simulink library "HANcoder_STM32_Target"  (R2018a)
settings: Solver=ode45  StartTime=0.0  StopTime=10.0  RelTol=1e-3  EnableMultiTasking=on
libraries: simulink x3
(part 3 of 7)

== system HANcoder_STM32_Target/STM32-E407/SPI ==
  SPI master init : Subsystem  Tag=HANcoder_TARGET_STM32_E407  mask(SPI master init){channel=SPI1: D13 & D12 & D11, speed=5250 kHz, polarity=Idle low, phase=Sample bit on 1st clock edge}
      mask prompts: speed "Communication speed"
      mask help:
      | Function
      | ==========
      | Initialized a SPI master channel.
      |
      | Parameters per channel
      | ======================
      | - Select channel
      | - Select communication speed
      | - Select clock signal polarity
      | - Select clock phase to sample a bit
      mask init:
      | spiChannelInfoStr = sfcn_spi_master_init_mcb(2, channel, speed, polarity, phase);
      settings: CopyFcn=sfcn_spi_master_init_chk();  MoveFcn=drawLogos
      mask Help: web('sfcn_spi_master_init.html')
      mask TypeOptions channel: SPI1: D13 & D12 & D11 | SPI2: UEXT 9 & 7 & 8
      mask Callback channel: sfcn_spi_master_init_chk();
      mask TypeOptions speed: 21000 kHz | 10500 kHz | 5250 kHz | 2625 kHz | 1312.5 kHz | 656.25 kHz | 328.125 kHz | 164.0625 kHz
      mask TypeOptions polarity: Idle low | Idle high
      mask TypeOptions phase: Sample bit on 1st clock edge | Sample bit on 2nd clock edge
      mask Display: fprintf('SPI master init\n%s', spiChannelInfoStr);patch([211 217 217],[8 14 2],[1 0 0]);patch([219 219 225],[14 2 8],[0 0 0.35]);
  SPI master transfer : Subsystem  Tag=HANcoder_TARGET_STM32_E407  mask(SPI master transfer){channel=SPI1: D13 & D12 & D11, useSS=off, SSpin=CON2 - A0, SSenable=on, SSdisable=on, delayCycles=0, tsamp=-1}
      mask prompts: useSS "Use slave select output"; SSpin "Slave select output pin"; SSenable "Enable slave select before transfer"; SSdisable "Disable slave select after transfer"; delayCycles "Delay cycles between slave select enable and transfer"; tsamp "Sample time"
      mask help:
      | Function
      | ==========
      | Performs a byte transfer via SPI.
      |
      | Parameters per channel
      | ======================
      | - Select channel
      | - Select if a Slave Select output should be controlled
      |   * Select the Slave Select digital output pin
      |   * Select if the Slave Select should be made logic low before the transfer
      |   * Select if the Slave Select should be made logic high after the transfer
      |   * Enter the number of CPU cycles to delay between Slave Select enable and the transfer
      |
      | Inputs
      | ======
      | The byte value to send to the slave.
      |
      | Outputs
      | =======
      | The byte value received from the slave.
      mask init:
      | spiChannelInfoStr = sfcn_spi_master_transfer_mcb(2, channel, useSS, SSpin, SSenable, SSdisable, delayCycles);
      settings: MoveFcn=drawLogos
      mask Help: web('sfcn_spi_master_transfer.html')
      mask TypeOptions channel: SPI1: D13 & D12 & D11 | SPI2: UEXT 9 & 7 & 8
      mask TypeOptions SSpin: CON2 - A0 | CON2 - A1 | CON2 - A2 | CON2 - A3 | CON2 - A4 | CON2 - A5 | CON3 - D0 | CON3 - D1 | CON3 - D2 | CON3 - D3 | CON3 - D4 | CON3 - D5 | CON3 - D6 | CON3 - D7 | CON4 - D8 | CON4 - D9 | CON4 - D10 | CON4 - D11 | CON4 - D12 | CON4 - D13 | CON PD - 3 | CON PD - 4 | CON PD - 5 | CON PD - 6 | CON PD - 7 | CON PD - 8 | CON PD - 9 | CON PD - 10 | CON PD - 11 | CON PD - 12 | CON PD - 13 | CON PD - 14 | CON PD - 15 | CON PD - 16 | CON PD - 17 | CON PD - 18 | CON PE - 3 | CON PE - 4 | CON PE - 6 | CON PE - 10 | CON PE - 11 | CON PE - 12 | CON PE - 13 | CON PE - 14 | CON PE - 15 | CON PE - 16 | CON PE - 17 | CON PE - 18 | CON PF - 3 | CON PF - 4 | CON PF - 5 | CON PF - 6 | CON PF - 7 | CON PF - 8 | CON PF - 14 | CON PF - 15 | CON PF - 16 | CON PF - 17 | CON PF - 18 | CON PG - 3 | CON PG - 4 | CON PG - 5 | CON PG - 6 | CON PG - 7 | CON PG - 8 | CON PG - 9 | CON PG - 12 | CON PG - 13 | CON PG - 14 | CON PG - 16 | CON PG - 17
      mask Display: fprintf('SPI master transfer\n%s', spiChannelInfoStr);patch([210 216 216],[8 14 2],[1 0 0]);patch([218 218 224],[14 2 8],[0 0 0.35]);

== system HANcoder_STM32_Target/STM32-E407/System Config ==
  Base Sample Time config : Subsystem  Tag=HANcoder_TARGET_STM32_E407  Description=HANcoder Target STM32-E407 blockset version 0.5  mask(Base Sample Time config){baseSampleTime=10, extraStack=100}
      mask prompts: baseSampleTime "Define the base sample time [ms]"; extraStack "Additional task stack (bytes):"
      mask help:
      | Function
      | ==========
      | Sets the Base Sample Time in the model, and automatically sets the sample
      | time in the solver step time menu when the model is simulated or build.
      |
      | Parameters
      | ==========
      | Base Sample Time [milliseconds]
      | Default:    10[ms]
      | Min:        0.1[ms]
      |
      | Note: This is the only block where sample time is set in miliseconds,
      | all other blocks work with sample time in seconds
      |
      | It is possible to reserve extra stack space for the OS task that executes
      | the model on the embedded target (AppCtrlTask).
      mask init:
      | sfcn_base_sample_time_mcb(baseSampleTime*1000, extraStack, 2);
      | HANcoderStruct = get_param(gcb,'UserData');
      | BlocksetVersion = HANcoderStruct.BlocksetVersion;
      settings: MoveFcn=drawLogos
      mask Help: web('sfcn_base_sample_time.html')
      mask Display: fprintf('Blockset version %s\nBase Sample Time:\n %gms',BlocksetVersion,baseSampleTime);patch([91 97 97],[8 14 2],[1 0 0]);patch([99 99 105],[14 2 8],[0 0 0.35]);
  Build settings : Subsystem  Tag=HANcoder_TARGET_STM32_E407  mask(Build Settings){AutoASAP2add=on, AutoFlash=USB}
      mask prompts: AutoASAP2add "Add signals and parameters automatically"; AutoFlash "Automatic flash after build"
      mask help:
      | Function
      | ==========
      | Auto Add:
      | Here you can turn the automatic adding of Signals and Parameters on or off. If the option is on all the parameters and signals which are not defined in the workspace will be added. You will be prompted for the value.
      |
      | Auto Flash:
      | This option will automatically start MicroBoot with the selected interface.
      settings: MoveFcn=drawLogos
      mask Help: web('build_settings.html')
      mask TypeOptions AutoASAP2add: on | off
      mask TypeOptions AutoFlash: off | USB | CAN | Ethernet
      mask DialogControl ParameterTabVar0 Prompt: Auto Add
      mask DialogControl Control3 Prompt: With this option the undefined parameters and signals will automatically be added to the workspace for use with HANtune. You will be prompted for the parameter values.
      mask DialogControl ParameterTabVar01 Prompt: Auto Flash
      mask DialogControl Control2 Prompt: With this option you can choose to automatically start MicroBoot after the build is complete. MicroBoot will start flashing using the selected interface.
      mask Display: fprintf('Build settings\nAuto Add: %s\nAuto Flash: %s',AutoASAP2add, AutoFlash);patch([114 120 120],[8 14 2],[1 0 0]);patch([122 122 128],[14 2 8],[0 0 0.35]);
  CAN config : Subsystem  Tag=HANcoder_TARGET_STM32_E407  mask(CAN config){txBufSize=64, evBufSize=64, canBus1=off, baudRate1=500, rxMask1=hex2dec('00000000'), rxCode1=hex2dec('00000000'), rxMode1=Receive only 11-bit message identifiers, canBus2=off, baudRate2=500, rxMask2=hex2dec('00000000'), rxCode2=hex2dec('00000000'), rxMode2=Receive only 11-bit message identifiers}
      mask prompts: txBufSize "Transmit buffer size CAN bus (max 512)"; evBufSize "Event buffer size CAN bus"; canBus1 "Use CAN bus 1"; baudRate1 "Baudrate CAN bus 1 (kbit/s)"; rxMask1 "Reception filter Mask CAN bus 1"; rxCode1 "Reception filter Code CAN bus 1"; rxMode1 "Reception filter Mode CAN bus 1"; canBus2 "Use CAN bus 2"; baudRate2 "Baudrate CAN bus 2 (kbit/s)"; rxMask2 "Reception filter Mask CAN bus 2"; rxCode2 "Reception filter Code CAN bus 2"; rxMode2 "Reception filter Mode CAN bus 2"
      mask help:
      | Function
      | ==========
      | Configures the settings for the STM32's CAN busses.
      |
      | Pinout
      | ==========
      | CAN1:   RX: CON PD - 3
      |             TX: CON PD - 4
      | CAN2:   RX: CON4 - D11
      |             TX: CON3 -  D1
      |
      | Parameters per channel
      | ======================
      | - Activate channel
      | - Select baud rate (default 500[kbit/s])
      | - Select reception acceptance filter Code
      | - Select reception acceptance filter Mask
      | - Select reception acceptance filter Mode
      mask init:
      | sfcn_can_config_mcb(txBufSize, evBufSize, canBus1, baudRate1, rxMask1, rxCode1, rxMode1, canBus2, baudRate2, rxMask2, rxCode2, rxMode2);
      settings: MoveFcn=drawLogos
      mask Help: web('sfcn_can_config.html')
      mask TypeOptions baudRate1: 125 | 250 | 500 | 1000
      mask TypeOptions rxMode1: Receive only 11-bit message identifiers | Receive only 29-bit message identifiers | Received both 11- and 29-bit message identifiers
      mask TypeOptions baudRate2: 125 | 250 | 500 | 1000
      mask TypeOptions rxMode2: Receive only 11-bit message identifiers | Receive only 29-bit message identifiers | Received both 11- and 29-bit message identifiers
      mask Display: fprintf('CAN1 : %x\nCAN2 : %x',canBus1, canBus2);patch([67 73 73],[8 14 2],[1 0 0]);patch([75 75 81],[14 2 8],[0 0 0.35]);
  Custom ID config : Subsystem  Tag=HANcoder_TARGET_STM32_E407  mask(Custom ID config){softID=softwareID, softNUM=1}
      mask prompts: softID "Software ID Name"; softNUM "Software Version Number"
      mask help:
      | Function:
      | =========
      | This block can be used to override the generated software ID as the current software version which is used for identification purposes.
      | It can also be used to add a version number behind the software ID.
      |
      | Details:
      | ========
      | If only a software version number is filled in, a software ID will be generated and the version number will be placed behind it.
      | Atleast one pf the fields has to be filled in.
      |
      | Parameters:
      | ===========
      | Software ID name:
      | Fill in the desired custom ID. Must fit in a UINT8
      | Software Version Number:
      | Fill in the desired version number. Must fit in a UINT8
      mask init:
      | sfcn_custom_version_config_mcb(softID, softNUM)
      settings: MoveFcn=drawLogos
      mask Help: web('sfcn_custom_ID_config.html')
      mask Display: fprintf('Custom software ID:\n "%s"\n Software version:\n "%s"', char(softID), char(softNUM));patch([112 118 118],[8 14 2],[1 0 0]);patch([120 120 126],[14 2 8],[0 0 0.35]);
  Ethernet config : Subsystem  Tag=HANcoder_TARGET_STM32_E407  mask(Ethernet config){ip1=169, ip2=254, ip3=19, ip4=63, nm1=255, nm2=255, nm3=0, nm4=0, gw1=169, gw2=254, gw3=1, gw4=1}
      mask prompts: ip1 "IP address 1"; ip2 "IP address 2"; ip3 "IP address 3"; ip4 "IP address 4"; nm1 "Netmask 1"; nm2 "Netmask 2"; nm3 "Netmask 3"; nm4 "Netmask 4"; gw1 "Gateway address 1"; gw2 "Gateway address 2"; gw3 "Gateway address 3"; gw4 "Gateway address 4"
      mask help:
      | Function
      | ==========
      | Configures the settings for the STM32's Ethernet interface.
      |
      | Parameters
      | ======================
      | - IP address
      | - Network mask
      | - Gateway address
      mask init:
      | sfcn_ethernet_config_mcb(ip1, ip2, ip3, ip4, nm1, nm2, nm3, nm4, gw1, gw2, gw3, gw4)
      settings: MoveFcn=drawLogos
      mask Help: web('sfcn_ethernet_config.html')
      mask Display: fprintf('Ethernet config');patch([68 74 74],[8 14 2],[1 0 0]);patch([76 76 82],[14 2 8],[0 0 0.35]);
  XCP on CAN config : Subsystem  Tag=HANcoder_TARGET_STM32_E407  mask(XCP on CAN config){canBus=CAN 1, croID=hex2dec('665'), dtoID=hex2dec('666')}
      mask prompts: canBus "CAN channel"; croID "CRO identifier"; dtoID "DTO identifier"
      mask help:
      | Function
      | ==========
      | Implements XCP communication into your application using the CAN network.
      |
      | Parameter
      | ==========
      | Specify the CAN channel to be used for XCP.
      | Specify the CAN CRO message identifier for XCP (master->slave).
      | Specify the CAN DTO message identifier for XCP (slave->master).
      |
      | Notes
      | ==========
      | Baudrates can be modified in the CAN config block.
      mask init:
      | sfcn_can_xcp_config_mcb(canBus, croID, dtoID)
      settings: MoveFcn=drawLogos
      mask Help: web('sfcn_can_xcp_config.html')
      mask TypeOptions canBus: CAN 1 | CAN 2
      mask Display: fprintf('XCP over CAN: %x',canBus);patch([69 75 75],[8 14 2],[1 0 0]);patch([77 77 83],[14 2 8],[0 0 0.35]);
  XCP on TCP/IP config : Subsystem  Tag=HANcoder_TARGET_STM32_E407  mask(XCP on TCP/IP config){port=1000}
      mask prompts: port "TCP/IP port"
      mask help:
      | Function
      | ==========
      | Implements XCP communication into your application using TCP/IP.
      |
      | Parameter
      | ==========
      | Specify the TCP/IP port to listen on for XCP.
      |
      | Notes
      | ==========
      | Requires the Ethernet config block to be present in the model.
      mask init:
      | sfcn_tcpip_xcp_config_mcb(port)
      settings: MoveFcn=drawLogos
      mask Help: web('sfcn_tcpip_xcp_config.html')
      mask Display: fprintf('XCP on TCP/IP');patch([69 75 75],[8 14 2],[1 0 0]);patch([77 77 83],[14 2 8],[0 0 0.35]);
  XCP on USB config : Subsystem  Tag=HANcoder_TARGET_STM32_E407  mask(XCP on USB config){}
      mask help:
      | Function
      | ==========
      | Implements XCP communication into your application using the USB Virtual COM-port.
      | This functionality is available on the USB OTG1 connector on the board.
      mask init:
      | sfcn_usb_xcp_config_mcb()
      settings: MoveFcn=drawLogos
      mask Help: web('sfcn_usb_xcp_config.html')
      mask Display: fprintf('XCP over USB');patch([69 75 75],[8 14 2],[1 0 0]);patch([77 77 83],[14 2 8],[0 0 0.35]);

== system HANcoder_STM32_Target/STM32-E407/System Management ==
  Enter Critical Section : Subsystem  Tag=HANcoder_TARGET_STM32_E407  mask(Enter a critical section){tsamp=-1}
      mask prompts: tsamp "Sample time"
      mask help:
      | Function
      | ==========
      | Enters a critical section that can not be interrupted. This block must
      | always be used in a pair together with "Exit Critical Section". Click the
      | Help-button for a detailed example on how to use this block.
      mask init:
      | sfcn_critical_enter_mcb();
      settings: MoveFcn=drawLogos
      mask Help: web('sfcn_critical_section.html');
      mask Display: fprintf('Enter Critical Section');patch([95 101 101],[8 14 2],[1 0 0]);patch([103 103 109],[14 2 8],[0 0 0.35]);
  Exit Critical Section : Subsystem  Tag=HANcoder_TARGET_STM32_E407  mask(Exit a critical section){tsamp=-1}
      mask prompts: tsamp "Sample time"
      mask help:
      | Function
      | ==========
      | Exits a critical section. This block must always be used in a pair together
      | with "Enter Critical Section". Click the Help-button for a detailed example
      | on how to use this block.
      mask init:
      | sfcn_critical_exit_mcb();
      settings: MoveFcn=drawLogos
      mask Help: web('sfcn_critical_section.html');
      mask Display: fprintf('Exit Critical Section');patch([95 101 101],[8 14 2],[1 0 0]);patch([103 103 109],[14 2 8],[0 0 0.35]);
  Get CPU load : Subsystem  Tag=HANcoder_TARGET_STM32_E407  mask(Get CPU load){mode=Current CPU load, tsamp=-1}
      mask prompts: tsamp "Sample time"
      mask help:
      | Function
      | ==========
      | Get the CPU load of the system.
      |
      | Parameters
      | ==========
      | Mode specifies if the current CPU load should be read or the maximum CPU
      | load since reset.
      |
      | Outport
      | ==========
      | CPU load as a percentage.
      mask init:
      | if mode==1
      |   modeStr = 'current';
      | else
      |   modeStr = 'maximum';
      | end
      | sfcn_controller_cpu_getload_mcb(mode);
      settings: MoveFcn=drawLogos
      mask Help: web('sfcn_controller_cpu_getload.html');
      mask TypeOptions mode: Current CPU load | Maximum CPU load
      mask Display: fprintf('Get %s\nCPU load', modeStr);patch([95 101 101],[8 14 2],[1 0 0]);patch([103 103 109],[14 2 8],[0 0 0.35]);
  Get free Heap : Subsystem  Tag=HANcoder_TARGET_STM32_E407  mask(Get free Heap){tsamp=-1}
      mask prompts: tsamp "Sample time"
      mask help:
      | Function
      | ==========
      | Obtains the number of bytes that are still available on the heap.
      |
      | Outport
      | ==========
      | Number of bytes that are still available on the heap.
      mask init:
      | sfcn_controller_getheap_mcb();
      settings: MoveFcn=drawLogos
      mask Help: web('sfcn_controller_getheap.html');
      mask Display: fprintf('Get free Heap');patch([95 101 101],[8 14 2],[1 0 0]);patch([103 103 109],[14 2 8],[0 0 0.35]);
  Get free Stack : Subsystem  Tag=HANcoder_TARGET_STM32_E407  mask(Get free Stacl){taskIdx=Application Control Task, tsamp=-1}
      mask prompts: taskIdx "Task name"; tsamp "Sample time"
      mask help:
      | Function
      | ========
      | Obtains the number of bytes that are still available on the stack of a particular task.
      |
      | Parameter
      | =========
      | Name of the task for which the free stack space should be read.
      |
      | Outport
      | =======
      | Number of bytes that are still available on the task's stack.
      mask init:
      | sfcn_controller_getstack_mcb(taskIdx);
      settings: MoveFcn=drawLogos
      mask Help: web('sfcn_controller_getstack.html');
      mask TypeOptions taskIdx: Idle Task | Timer Task | Can Event Task | Can Transmit Task | Application Control Task | Measurement and Calibration Network Task | Ethernet Interface Task | Ethernet Link Task | TCP/IP Task | File Logger Task | CANopen Node Task | ADC Conversion Task
      mask Display: fprintf('Get free Stack');patch([95 101 101],[8 14 2],[1 0 0]);patch([103 103 109],[14 2 8],[0 0 0.35]);
  Reset ECU : Subsystem  Tag=HANcoder_TARGET_STM32_E407  mask(Reset ECU){}
      mask help:
      | Function
      | ==========
      | Triggering this block causes the ECU to reset.
      mask init:
      | sfcn_controller_reset_mcb()
      settings: MoveFcn=drawLogos
      mask Help: web('sfcn_controller_reset.html');
      mask Display: fprintf('Reset ECU');patch([60 66 66],[8 14 2],[1 0 0]);patch([68 68 74],[14 2 8],[0 0 0.35]);

== system HANcoder_STM32_Target/STM32-E407/Timer Inputs ==
  Quadrature Encoder Get : Subsystem  Tag=HANcoder_TARGET_STM32_E407  mask(Quadrature Encoder Inputs){moduleID=TIM1: CON PE - 12 & 14 (5V Tolerant), config=Floating, counterReset=off, tsamp=-1}
      mask prompts: moduleID "Quad encoder module"; config "Configuration"; counterReset "Show counter reset input"; tsamp "Sample time"
      mask help:
      | Function
      | ========
      | Reads the counter of the quadrature encoder module.
      |
      | Parameters
      | ==========
      | Quadrature encoder module:
      |   Selects the quadrature encoder module. The channel A and B signals of the
      |   encoder should be connected to the 2 input pins that belong to the module.
      |
      | Configuration:
      |   Determines if the input is floating or is connected to an internal
      |   pull-up or pull-down resistor.
      |
      | Show counter reset input:
      |   Configures if the input port for the counter reset should be shown.
      |
      |
      | Outport
      | ==========
      | 32-bit signed counter. The counter starts at zero and counts up or down
      | depending on the direction of the motor.
      mask init:
      | moduleIDInfoStr = sfcn_quad_encoder_get_mcb(2,moduleID, counterReset, config);
      settings: CopyFcn=sfcn_quad_encoder_get_chk();  MoveFcn=drawLogos
      mask Help: web('sfcn_quad_encoder_get.html');
      mask TypeOptions moduleID: TIM1: CON PE - 12 & 14 (5V Tolerant) | TIM3: CON4 - D12 & D11 (5V Tolerant) | TIM4: CON PD - 15 & 16 (5V Tolerant) | TIM8: UEXT - 3 & 4 (5V Tolerant)
      mask Callback moduleID: sfcn_quad_encoder_get_chk();
      mask TypeOptions config: Floating | Pullup | Pulldown
      mask Display: fprintf('Quad Encoder Get\n%s', moduleIDInfoStr);patch([135 141 141],[8 14 2],[1 0 0]);patch([143 143 149],[14 2 8],[0 0 0.35]);
  Timer Input Get : Subsystem  Tag=HANcoder_TARGET_STM32_E407  mask(Timer Input Get){pin=TIM1: CON PE - 12 - 5V Tolerant, zeroHzTimeoutMs=2000, tsamp=-1}
      mask prompts: pin "Timer input pin"; zeroHzTimeoutMs "0 Hz detection time (ms)"; tsamp "Sample time"
      mask help:
      | Function
      | ========
      | Reads the information from a timer input pin.
      |
      | Parameters
      | ==========
      | Timer input pin:
      |   Selects the timer input pin.
      |
      | Zero Hz detection time:
      |   Determines after how many milliseconds since the last edge the 0 Hz
      |   detected output flag should go high.
      |
      | Outport
      | ==========
      | Frequency
      |   The last measured frequency on the pin in Hz.
      |
      | Duty cycle
      |   The last measured duty cycle on the pin as a % with a scaling factor of 100 for
      |   improved resolution. So 5000 = 50% for example.
      |
      | Edge count
      |   The number of edges that were detected on the input pin since startup.
      |
      | Edge timestamp
      |   A 32-bit timestamp value of the last edge. The timestamp is derived from an
      |   internal 32-bit free running counter that runs at 21 Mhz.
      |
      | 0 Hz detected
      |   A boolean flag that will go high if no edges were detected for the time specified
      |   as the zero Hz detection time. Upon the next edge the flag will go low again.
      mask init:
      | timeinPinIdInfoStr = sfcn_timein_get_mcb(2, pin, zeroHzTimeoutMs);
      settings: CopyFcn=sfcn_timein_get_chk();  MoveFcn=drawLogos
      mask Help: web('sfcn_timein_get.html');
      mask TypeOptions pin: TIM1: CON PE - 12 - 5V Tolerant | TIM1: CON PE - 14 - 5V Tolerant | TIM1: CON PE - 16 - 5V Tolerant | TIM1: CON PE - 17 - 5V Tolerant | TIM2: CON4 - D13 | TIM3: CON4 - D12 - 5V Tolerant | TIM3: CON4 - D11 - 5V Tolerant | TIM4: CON PD - 15 - 5V Tolerant | TIM4: CON PD - 16 - 5V Tolerant | TIM8: UEXT - 3 - 5V Tolerant | TIM8: UEXT - 4 - 5V Tolerant | TIM9: CON3 - D4 - 5V Tolerant | TIM9: CON3 - D5 - 5V Tolerant | TIM10: CON PF - 9 -  5V Tolerant | TIM11: CON PF - 10 -  5V Tolerant | TIM13: CON PF - 11 -  5V Tolerant | TIM14: CON PF - 12 -  5V Tolerant
      mask Callback pin: sfcn_timein_get_chk();
      mask Display:
      | fprintf('Timer Input Get\n%s', timeinPinIdInfoStr);
      | port_label('output', 1, 'Frequency');
      | port_label('output', 2, 'Duty cycle');
      | port_label('output', 3, 'Edge count');
      | port_label('output', 4, 'Edge state');
      | port_label('output', 5, 'Edge timestamp');
      | port_label('output', 6, 'Counter timestamp');
      | port_label('output', 7, '0 Hz detected');patch([255 261 261],[8 14 2],[1 0 0]);patch([263 263 269],[14 2 8],[0 0 0.35]);
  Timer Input IRQ : Subsystem  Tag=HANcoder_TARGET_STM32_E407  mask(Timer Input IRQ){pin=TIM1 CON PE - 12 - 5V Tolerant}
      mask prompts: pin "Timer input pin"
      mask help:
      | Function
      | ========
      | Enables a function call subsystem to be connected that is executed on interrupt level
      | each time an edge change on the input pin was detected.
      |
      | Parameters
      | ==========
      | Timer input pin:
      |   Selects the timer input pin.
      |
      | Outport
      | =======
      | IRQ
      |   Allows connection of a function call subsystem.
      |   (This function call subsystem cannot be empty!)
      mask init:
      | timeinPinIdInfoStr = sfcn_timein_irq_mcb(2, pin);
      settings: CopyFcn=sfcn_timein_irq_chk();  MoveFcn=drawLogos
      mask Help: web('sfcn_timein_irq.html');
      mask TypeOptions pin: TIM1 CON PE - 12 - 5V Tolerant | TIM1 CON PE - 14 - 5V Tolerant | TIM1 CON PE - 16 - 5V Tolerant | TIM1 CON PE - 17 - 5V Tolerant | TIM2 CON4 - D13 | TIM3 CON4 - D12 - 5V Tolerant | TIM3 CON4 - D11 - 5V Tolerant | TIM4 CON PD - 15 - 5V Tolerant | TIM4 CON PD - 16 - 5V Tolerant | TIM8 UEXT - 3 - 5V Tolerant | TIM8 UEXT - 4 - 5V Tolerant | TIM9 CON3 - D4 - 5V Tolerant | TIM9 CON3 - D5 - 5V Tolerant | TIM10 CON PF - 9 - 5V Tolerant | TIM11 CON PF - 10 - 5V Tolerant | TIM13 CON PF - 11 - 5V Tolerant | TIM14 CON PF - 12 - 5V Tolerant
      mask Callback pin: sfcn_timein_irq_chk();
      mask Display: fprintf('Timer Input IRQ\n%s', timeinPinIdInfoStr);patch([155 161 161],[8 14 2],[1 0 0]);patch([163 163 169],[14 2 8],[0 0 0.35]);

== system HANcoder_STM32_Target/STM32-E407/Timer Outputs ==
  Compare Event IRQ : Subsystem  Tag=HANcoder_TARGET_STM32_E407  mask(Compare Event IRQ){pin=TIM1 - CON PE - 12 - 5V Tolerant}
      mask prompts: pin "Timer output pin"
      mask help:
      | Function
      | ========
      | Enables a function call subsystem to be connected that is executed on interrupt
      | level each time an output compare event was triggered.
      |
      | Parameters
      | ==========
      | Timer Output Pin:
      |   Selects the timer channel.
      |
      | Outport
      | =======
      | IRQ
      |   Allows connection of a function call subsystem.
      mask init:
      | timeoutPinIdInfoStr = sfcn_timeout_event_irq_mcb(2, pin);
      settings: CopyFcn=sfcn_timeout_event_irq_chk();  MoveFcn=drawLogos
      mask Help: web('sfcn_timeout_event_irq.html');
      mask TypeOptions pin: TIM1 - CON PE - 12 - 5V Tolerant | TIM1 - CON PE - 14 - 5V Tolerant | TIM1 - CON PE - 16 - 5V Tolerant | TIM1 - CON PE - 17 - 5V Tolerant | TIM2 - CON4 - D13 | TIM3 - CON4 - D12 - 5V Tolerant | TIM3 - CON4 - D11 - 5V Tolerant | TIM4 - CON PD - 15 - 5V Tolerant | TIM4 - CON PD - 16 - 5V Tolerant | TIM8 - UEXT - 3 - 5V Tolerant | TIM8 - UEXT - 4 - 5V Tolerant | TIM9 - CON3 - D4 - 5V Tolerant | TIM9 - CON3 - D5 - 5V Tolerant | TIM10 - CON PF - 9 - 5V Tolerant | TIM11 - CON PF - 10 - 5V Tolerant | TIM13 - CON PF - 11 - 5V Tolerant | TIM14 - CON PF - 12 - 5V Tolerant
      mask Callback pin: sfcn_timeout_event_irq_chk();
      mask Display: fprintf('Compare Event IRQ\n%s', timeoutPinIdInfoStr);patch([135 141 141],[8 14 2],[1 0 0]);patch([143 143 149],[14 2 8],[0 0 0.35]);
  Get Free Running Counter : Subsystem  Tag=HANcoder_TARGET_STM32_E407  mask(Get Free Running Counter){moduleID=TIM1 - CON PE - 12 & 14 & 16 & 17, tsamp=-1}
      mask prompts: moduleID "Timer module"; tsamp "Sample time"
      mask help:
      | Function
      | ========
      | Reads the timer module's internal 16-bit free running counter value.
      |
      | Parameters
      | ==========
      | Timer Module:
      |   Selects the timer module.
      |
      | Outport
      | =======
      | 16-bit free running counter value.
      mask init:
      | moduleIDInfoStr = sfcn_timeout_getrunningcounter_mcb(2, moduleID);
      settings: MoveFcn=drawLogos
      mask Help: web('sfcn_timeout_getrunningcounter.html');
      mask TypeOptions moduleID: TIM1 - CON PE - 12 & 14 & 16 & 17 | TIM2 - CON4 - D13 & n/a & n/a & n/a | TIM3 - CON4 - D12 & D11 & n/a & n/a | TIM4 - CON PD - 15 & 16 &n/a & n/a | TIM8 - UEXT - 3 & 4 & n/a & n/a | TIM9 - CON3 - D4 & D5 or PE - 8 & 9 | TIM10 - CON2 - A1 or CON PF - 9 | TIM11 - CON2 - A2 or CON PF - 10 | TIM13 - CON2 - A3 or CON PF - 11 | TIM14 - CON2 - A4 or CON PF - 12
      mask Display: fprintf('Get Free Running Counter\n%s', moduleIDInfoStr);patch([135 141 141],[8 14 2],[1 0 0]);patch([143 143 149],[14 2 8],[0 0 0.35]);
  Get Last Event Counter : Subsystem  Tag=HANcoder_TARGET_STM32_E407  mask(Get Last Event Counter){pin=TIM1 - CON PE - 12 - 5V Tolerant, tsamp=-1}
      mask prompts: pin "Timer output pin"; tsamp "Sample time"
      mask help:
      | Function
      | ========
      | Reads the timer channel's timestamp of the 16-bit free running counter
      | value at which the last output compare event occurred.
      |
      | Parameters
      | ==========
      | Timer Output Pin:
      |   Selects the timer channel.
      |
      | Outport
      | =======
      | 16-bit free running counter timestamp of the last output compare event.
      mask init:
      | timeoutPinIdInfoStr = sfcn_timeout_getlasteventcounter_mcb(2, pin);
      settings: MoveFcn=drawLogos
      mask Help: web('sfcn_timeout_getlasteventcounter.html');
      mask TypeOptions pin: TIM1 - CON PE - 12 - 5V Tolerant | TIM1 - CON PE - 14 - 5V Tolerant | TIM1 - CON PE - 16 - 5V Tolerant | TIM1 - CON PE - 17 - 5V Tolerant | TIM2 - CON4 - D13 | TIM3 - CON4 - D12 - 5V Tolerant | TIM3 - CON4 - D11 - 5V Tolerant | TIM4 - CON PD - 15 - 5V Tolerant | TIM4 - CON PD - 16 - 5V Tolerant | TIM8 - UEXT - 3 - 5V Tolerant | TIM8 - UEXT - 4 - 5V Tolerant | TIM9 - CON3 - D4 - 5V Tolerant | TIM9 - CON3 - D5 - 5V Tolerant | TIM10 - CON PF - 9 - 5V Tolerant | TIM11 - CON PF - 10 - 5V Tolerant | TIM13 - CON PF - 11 - 5V Tolerant | TIM14 - CON PF - 12 - 5V Tolerant
      mask Display: fprintf('Get Last Event Counter\n%s', timeoutPinIdInfoStr);patch([135 141 141],[8 14 2],[1 0 0]);patch([143 143 149],[14 2 8],[0 0 0.35]);
  Output Compare Init : Subsystem  Tag=HANcoder_TARGET_STM32_E407  mask(Output Compare Init){moduleID=TIM1 - CON PE - 12 & 14 & 16 & 17, frequency=2000000, enableIRQoutput=off}
      mask prompts: moduleID "Timer module"; frequency "Frequency (free running counter) [Hz]"; enableIRQoutput "Enable IRQ output"
      mask help:
      | Function
      | ========
      | Initializes the timer module to allow output compare functionality on the
      | module's channels.
      |
      | Parameters
      | ==========
      | Timer Module:
      |   Selects the timer module.
      |
      | Frequency:
      |   Frequency at which the 16-bit free running counter counts.
      |
      | Enable IRQ output
      |   Controls whether or not the IRQ output is available.
      |
      | Outport
      | =======
      | IRQ
      |   Allows connection of a function call subsystem for the free running
      |   counter overflow event.
      mask init:
      | moduleIDInfoStr = sfcn_timeout_init_mcb(2, moduleID, frequency, enableIRQoutput);
      settings: CopyFcn=sfcn_timeout_init_chk();  MoveFcn=drawLogos
      mask Help: web('sfcn_timeout_init.html');
      mask TypeOptions moduleID: TIM1 - CON PE - 12 & 14 & 16 & 17 | TIM2 - CON4 - D13 & n/a & n/a & n/a | TIM3 - CON4 - D12 & D11 & n/a & n/a | TIM4 - CON PD - 15 & 16 &n/a & n/a | TIM8 - UEXT - 3 & 4 & n/a & n/a | TIM9 - CON3 - D4 & D5 or PE - 8 & 9 | TIM10 - CON2 - A1 or CON PF - 9 | TIM11 - CON2 - A2 or CON PF - 10 | TIM13 - CON2 - A3 or CON PF - 11 | TIM14 - CON2 - A4 or CON PF - 12
      mask Callback moduleID: sfcn_timeout_init_chk();
      mask Display: fprintf('Output Compare Init\n%s', moduleIDInfoStr);patch([135 141 141],[8 14 2],[1 0 0]);patch([143 143 149],[14 2 8],[0 0 0.35]);
  Reset Free Running Counter : Subsystem  Tag=HANcoder_TARGET_STM32_E407  mask(Reset Free Running Counter){moduleID=TIM1 - CON PE - 12 & 14 & 16 & 17}
      mask prompts: moduleID "Timer module"
      mask help:
      | Function
      | ========
      | Resets the value of the timer module's 16-bit free running counter back to
      | 0.
      |
      | Triggerport
      | ===========
      | Connect the port to a trigger source to execute the block only when necessary.
      mask init:
      | moduleIDInfoStr = sfcn_timeout_resetcounter_mcb(2, moduleID);
      settings: MoveFcn=drawLogos
      mask Help: web('sfcn_timeout_resetcounter.html');
      mask TypeOptions moduleID: TIM1 - CON PE - 12 & 14 & 16 & 17 | TIM2 - CON4 - D13 & n/a & n/a & n/a | TIM3 - CON4 - D12 & D11 & n/a & n/a | TIM4 - CON PD - 15 & 16 &n/a & n/a | TIM8 - UEXT - 3 & 4 & n/a & n/a | TIM9 - CON3 - D4 & D5 or PE - 8 & 9 | TIM10 - CON2 - A1 or CON PF - 9 | TIM11 - CON2 - A2 or CON PF - 10 | TIM13 - CON2 - A3 or CON PF - 11 | TIM14 - CON2 - A4 or CON PF - 12
      mask Display: fprintf('Reset Free Running Counter\n%s', moduleIDInfoStr);patch([132 138 138],[8 14 2],[1 0 0]);patch([140 140 146],[14 2 8],[0 0 0.35]);
  Schedule Compare Event : Subsystem  Tag=HANcoder_TARGET_STM32_E407  mask(Schedule Compare Event){pin=TIM1 - CON PE - 12 - 5V Tolerant, tsamp=-1}
      mask prompts: pin "Timer output pin"; tsamp "Sample time"
      mask help:
      | Function
      | ========
      | Schedules the next output compare event. The first input determines the
      | value of the timer module's 16-bit free running counter when the event
      | should trigger. The second input determines the action that should
      | be taken on the timer channel's pin.
      |
      | Parameters
      | ==========
      | Timer output pin:
      |   Selects the timer channel's pin.
      |
      | Inport
      | ======
      | Counter
      |   Value of the timer module's 16-bit free running counter at which the
      |   event should trigger.
      |
      | Action
      |   Action to take on the channel's pin when the event triggers:
      |   0: set output pin to logic low.
      |   1: set output pin to logic high.
      |   2: invert logic state of the outpin pin.
      |   3: do nothing to the output pin.
      mask init:
      | timeoutPinIdInfoStr = sfcn_timeout_scheduleevent_mcb(2, pin);
      settings: MoveFcn=drawLogos
      mask Help: web('sfcn_timeout_scheduleevent.html');
      mask TypeOptions pin: TIM1 - CON PE - 12 - 5V Tolerant | TIM1 - CON PE - 14 - 5V Tolerant | TIM1 - CON PE - 16 - 5V Tolerant | TIM1 - CON PE - 17 - 5V Tolerant | TIM2 - CON4 - D13 | TIM3 - CON4 - D12 - 5V Tolerant | TIM3 - CON4 - D11 - 5V Tolerant | TIM4 - CON PD - 15 - 5V Tolerant | TIM4 - CON PD - 16 - 5V Tolerant | TIM8 - UEXT - 3 - 5V Tolerant | TIM8 - UEXT - 4 - 5V Tolerant | TIM9 - CON3 - D4 - 5V Tolerant | TIM9 - CON3 - D5 - 5V Tolerant | TIM10 - CON PF - 9 - 5V Tolerant | TIM11 - CON PF - 10 - 5V Tolerant | TIM13 - CON PF - 11 - 5V Tolerant | TIM14 - CON PF - 12 - 5V Tolerant
      mask Display: fprintf('Schedule Compare Event\n%s', timeoutPinIdInfoStr);patch([135 141 141],[8 14 2],[1 0 0]);patch([143 143 149],[14 2 8],[0 0 0.35]);

== system HANcoder_STM32_Target/STM32-E407/UART ==
  UART init : Subsystem  Tag=HANcoder_TARGET_STM32_E407  mask(UART init){channel=UART1: CON3 - D1 & D0, baudrate=19200, databits=8, parity=none, stopbits=1, txbufsize=32, rxbufsize=32, useStatusOut=off}
      mask prompts: baudrate "Baudrate (bit/s)"; txbufsize "Transmit buffer size"; rxbufsize "Receive buffer size"; useStatusOut "Use status output"
      mask help:
      | Function
      | ==========
      | Initialized a UART channel.
      |
      | Parameters per channel
      | ======================
      | - Select channel (TX & RX)
      | - Select baudrate
      | - Select number of databits
      | - Select parity
      | - Select number of stopbits
      | - Configure the size of the transmit buffer
      | - Configure the size of the reception buffer
      | - Enable/disable the status output port
      mask init:
      | uartChannelInfoStr = sfcn_uart_init_mcb(2, channel, baudrate, databits, parity, stopbits, txbufsize, rxbufsize, useStatusOut);
      settings: CopyFcn=sfcn_uart_init_chk();  MoveFcn=drawLogos
      mask Help: web('sfcn_uart_init.html')
      mask TypeOptions channel: UART1: CON3 - D1 & D0 | UART2: CON PD - 8 & 9 | UART3: CON PD - 11 & 12 | UART6: UEXT - 3 & 4
      mask Callback channel: sfcn_uart_init_chk();
      mask TypeOptions baudrate: 300 | 600 | 1200 | 2400 | 4800 | 9600 | 19200 | 38400 | 57600 | 115200
      mask TypeOptions databits: 8 | 9
      mask TypeOptions parity: none | even | odd
      mask TypeOptions stopbits: 1 | 2
      mask Display: fprintf('UART init\n%s', uartChannelInfoStr);patch([236 242 242],[8 14 2],[1 0 0]);patch([244 244 250],[14 2 8],[0 0 0.35]);
  UART receive : Subsystem  Tag=HANcoder_TARGET_STM32_E407  mask(UART receive){channel=UART1: CON3 - D1 & D0, useStatusOut=off, tsamp=-1}
      mask prompts: useStatusOut "Use status outport"; tsamp "Sample time"
      mask help:
      | Function
      | ==========
      | Reads a byte from the UART reception buffer.
      |
      | Parameters per channel
      | ======================
      | - Select channel (TX & RX)
      | - Select if the status output should be enabled.
      |
      | Outputs
      | =======
      | - The value of the receive byte.
      | - When the status output is 0, the reception buffer was empty.
      mask init:
      | uartChannelInfoStr = sfcn_uart_receive_mcb(2, channel, useStatusOut);
      settings: MoveFcn=drawLogos
      mask Help: web('sfcn_uart_receive.html')
      mask TypeOptions channel: UART1: CON3 - D1 & D0 | UART2: CON PD - 8 & 9 | UART3: CON PD - 11 & 12 | UART6: UEXT - 3 & 4
      mask Display: fprintf('UART receive\n%s', uartChannelInfoStr);patch([240 246 246],[8 14 2],[1 0 0]);patch([248 248 254],[14 2 8],[0 0 0.35]);
  UART receive buffer status : Subsystem  Tag=HANcoder_TARGET_STM32_E407  mask(UART receive buffer status){channel=UART1: CON3 - D1 & D0, tsamp=-1}
      mask prompts: tsamp "Sample time"
      mask help:
      | Function
      | ==========
      | Obtains the number of received bytes that are currently stored in the
      | reception buffer.
      |
      | Parameters per channel
      | ======================
      | - Select channel (TX & RX)
      |
      | Outputs
      | ======
      | - The number of bytes currently stored in the reception buffer.
      mask init:
      | uartChannelInfoStr = sfcn_uart_receive_size_mcb(2, channel);
      settings: MoveFcn=drawLogos
      mask Help: web('sfcn_uart_receive_size.html')
      mask TypeOptions channel: UART1: CON3 - D1 & D0 | UART2: CON PD - 8 & 9 | UART3: CON PD - 11 & 12 | UART6: UEXT - 3 & 4
      mask Display: fprintf('UART receive buffer status\n%s', uartChannelInfoStr);patch([245 251 251],[8 14 2],[1 0 0]);patch([253 253 259],[14 2 8],[0 0 0.35]);
  UART send : Subsystem  Tag=HANcoder_TARGET_STM32_E407  mask(UART send){channel=UART1: CON3 - D1 & D0, useStatusOut=off, tsamp=-1}
      mask prompts: useStatusOut "Use status outport"; tsamp "Sample time"
      mask help:
      | Function
      | ==========
      | Transmits a byte on the UART communication interface.
      |
      | Parameters per channel
      | ======================
      | - Select channel (TX & RX)
      | - Select if the status output should be enabled.
      |
      | Inputs
      | ======
      | - The byte to send
      |
      | Outputs
      | =======
      | - When the status output is 0, the byte could not be transmitted. Probably
      |   because the transmit buffer was configured too small.
      mask init:
      | uartChannelInfoStr = sfcn_uart_send_mcb(2, channel, useStatusOut);
      settings: MoveFcn=drawLogos
      mask Help: web('sfcn_uart_send.html')
      mask TypeOptions channel: UART1: CON3 - D1 & D0 | UART2: CON PD - 8 & 9 | UART3: CON PD - 11 & 12 | UART6: UEXT - 3 & 4
      mask Display: fprintf('UART send\n%s', uartChannelInfoStr);patch([245 251 251],[8 14 2],[1 0 0]);patch([253 253 259],[14 2 8],[0 0 0.35]);

== system HANcoder_STM32_Target/STM32-E407/UDP ==
  UDP Client Send : Subsystem  Tag=HANcoder_TARGET_STM32_E407  mask(UDP Client Send){ip1=192, ip2=168, ip3=178, ip4=35, port=2000, inputNumber=10, dataType=uint8, byteOrder=on, tsamp=-1}
      mask prompts: ip1 "IP address 1"; ip2 "IP address 2"; ip3 "IP address 3"; ip4 "IP address 4"; inputNumber "Input ports"; dataType "Input datatype"; byteOrder "Byte order: Checked = MSB first, unchecked = LSB first."; tsamp "Sample time"
      mask help:
      | Function
      | ========
      | Sends a data packet to the UDP server with the specified IP address on
      | the specified port.
      |
      | Parameters
      | ==========
      | IP address 1:   First quad of the UDP server's IP address.
      | IP address 2:   Second quad of the UDP server's IP address.
      | IP address 3:   Third quad of the UDP server's IP address.
      | IP address 4:   Fourth quad of the UDP server's IP address.
      | Port:           Port to send the data packet on.
      | Input ports:    The amount of input ports.
      | Input datatype: The datatype of the input ports.
      | Byte order:     Select MSB or LSB first.
      | Sample time:    -1 or divisible by base sample time [seconds].
      |
      | Input
      | =====
      | Port 1..32      UDP packet data.
      mask init:
      | sfcn_udp_client_send_mcb(ip1,ip2,ip3,ip4,port,inputNumber,dataType,byteOrder);
      settings: MoveFcn=drawLogos
      mask Help: web('sfcn_udp_client_send.html');
      mask TypeOptions inputNumber: 1 | 2 | 3 | 4 | 5 | 6 | 7 | 8 | 9 | 10 | 11 | 12 | 13 | 14 | 15 | 16 | 17 | 18 | 19 | 20 | 21 | 22 | 23 | 24 | 25 | 26 | 27 | 28 | 29 | 30 | 31 | 32
      mask TypeOptions dataType: int8 | uint8 | int16 | uint16 | int32 | uint32 | boolean
      mask Display: fprintf('UDP Client Send\n\nport: %d\nip: %d.%d.%d.%d', port, ip1, ip2, ip3, ip4);patch([125 131 131],[8 14 2],[1 0 0]);patch([133 133 139],[14 2 8],[0 0 0.35]);
  UDP Server Init : Subsystem  Tag=HANcoder_TARGET_STM32_E407  mask(UDP Server Init){port=2001}
      mask help:
      | Function
      | ========
      | Initializes the UDP server to listen for and receive data packets on the
      | specified port.
      |
      | Parameters
      | ==========
      | Port:           Port to listen on.
      mask init:
      | sfcn_udp_server_init_mcb(port);
      settings: MoveFcn=drawLogos
      mask Help: web('sfcn_udp_server_init.html');
      mask Display: fprintf('UDP Server Init\n\nport: %d', port);patch([128 134 134],[8 14 2],[1 0 0]);patch([136 136 142],[14 2 8],[0 0 0.35]);
  UDP Server New Data Available : Subsystem  Tag=HANcoder_TARGET_STM32_E407  mask(UDP Server New Data Available){tsamp=-1}
      mask prompts: tsamp "Sample time"
      mask help:
      | Function
      | ========
      | Checks if the UDP server has new data in its internal receive buffer. This
      | new data flag is set each time a data packet is received by the UDP server.
      | It is reset when the application reads data from the receive buffer.
      |
      | Parameters
      | ==========
      | Sample time:    -1 or divisible by base sample time [seconds].
      |
      | Outport
      | ==========
      | 1 if new data is available in the UDP server's receive buffer that hasn't
      | been read yet by the application, 0 otherwise.
      mask init:
      | sfcn_udp_server_new_mcb();
      settings: MoveFcn=drawLogos
      mask Help: web('sfcn_udp_server_new.html');
      mask Display: fprintf('UDP Server New\nData Available');patch([128 134 134],[8 14 2],[1 0 0]);patch([136 136 142],[14 2 8],[0 0 0.35]);
  UDP Server Receive : Subsystem  Tag=HANcoder_TARGET_STM32_E407  mask(UDP Server Receive){outputNumber=10, dataType=uint8, byteOrder=on, startIdx=1, tsamp=-1}
      mask prompts: outputNumber "Output ports"; dataType "Output datatype"; byteOrder "Byte order: Checked = MSB first, unchecked = LSB first."; startIdx "Start index"; tsamp "Sample time"
      mask help:
      | Function
      | ========
      | Reads data from the UDP server's internal receive buffer.
      |
      | Parameters
      | ==========
      | Output ports:    The amount of output ports.
      | Output datatype: The datatype of the output ports.
      | Byte order:      Select MSB or LSB first.
      | Start index:     Start index in the server's buffer to start reading from.
      | Sample time:     -1 or divisible by base sample time [seconds].
      |
      | Output
      | ======
      | Port 1..32       UDP received packet data.
      mask init:
      | sfcn_udp_server_receive_mcb(outputNumber, dataType, byteOrder, startIdx);
      settings: MoveFcn=drawLogos
      mask Help: web('sfcn_udp_server_receive.html');
      mask TypeOptions outputNumber: 1 | 2 | 3 | 4 | 5 | 6 | 7 | 8 | 9 | 10 | 11 | 12 | 13 | 14 | 15 | 16 | 17 | 18 | 19 | 20 | 21 | 22 | 23 | 24 | 25 | 26 | 27 | 28 | 29 | 30 | 31 | 32
      mask TypeOptions dataType: int8 | uint8 | int16 | uint16 | int32 | uint32 | boolean
      mask TypeOptions startIdx: 1 | 2 | 3 | 4 | 5 | 6 | 7 | 8 | 9 | 10 | 11 | 12 | 13 | 14 | 15 | 16 | 17 | 18 | 19 | 20 | 21 | 22 | 23 | 24 | 25 | 26 | 27 | 28 | 29 | 30 | 31 | 32
      mask Display: fprintf('UDP Server Receive');patch([130 136 136],[8 14 2],[1 0 0]);patch([138 138 144],[14 2 8],[0 0 0.35]);
  UDP Server Receive Size : Subsystem  Tag=HANcoder_TARGET_STM32_E407  mask(UDP Server Receive Size){tsamp=-1}
      mask prompts: tsamp "Sample time"
      mask help:
      | Function
      | ========
      | Reads the size in bytes of the last UDP packet that was received by the UDP
      | server and stored in its internal receive buffer.
      |
      | Parameters
      | ==========
      | Sample time:    -1 or divisible by base sample time [seconds].
      |
      | Outport
      | ==========
      | Number of bytes currently stored in the UDP server's receive buffer.
      mask init:
      | sfcn_udp_server_count_mcb();
      settings: MoveFcn=drawLogos
      mask Help: web('sfcn_udp_server_count.html');
      mask Display: fprintf('UDP Server Receive\n Size');patch([128 134 134],[8 14 2],[1 0 0]);patch([136 136 142],[14 2 8],[0 0 0.35]);
